simulink model "motor_control"  (R2019a)
settings: Solver=VariableStepAuto  StartTime=0.0  StopTime=10.0  RelTol=1e-3
settings Model: Creator=COMPUMARTS  LastModifiedBy=COMPUMARTS

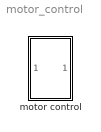
== system motor_control ==
  motor control : Subsystem

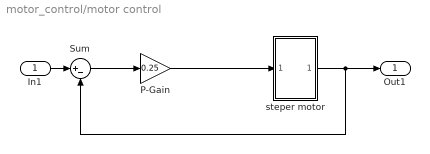
== system motor_control/motor control ==
  In1 : Inport
  P-Gain : Gain  Gain=0.25
  Sum : Sum  Inputs=|+-
  steper motor : Subsystem
  Out1 : Outport
  wires:
  P-Gain/1 -> steper motor/1(In1)
  Sum/1 -> P-Gain/1
  steper motor/1(Out1) -> Out1/1, Sum/2
  In1/1 -> Sum/1

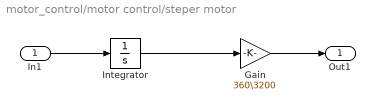
== system motor_control/motor control/steper motor ==
  In1 : Inport
  Gain : Gain  Gain=360\3200
  Integrator : Integrator
  Out1 : Outport
  wires:
  Integrator/1 -> Gain/1
  In1/1 -> Integrator/1
  Gain/1 -> Out1/1
